simulink model "untitled"  (R2017a)
settings: Solver=VariableStepAuto  StartTime=0.0  StopTime=10.0  RelTol=1e-3
settings Model: Creator=dskiee  LastModifiedBy=dskiee

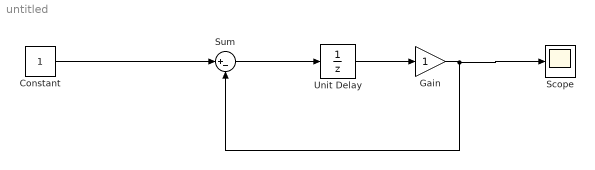
== system untitled ==
  Constant : Constant
  Gain : Gain
  Scope : Scope
  Sum : Sum  Inputs=|+-
  Unit Delay : UnitDelay  SampleTime=-1
  wires:
  Constant/1 -> Sum/1
  Gain/1 -> Scope/1, Sum/2
  Sum/1 -> Unit Delay/1
  Unit Delay/1 -> Gain/1
